simulink model "LQG_test"  (R2015a)
settings: Solver=ode5  StartTime=0.0  StopTime=10  FixedStep=5e-5  RelTol=1e-3
values from neighbouring files (symbols this model uses):
  Ak = [-152.325686755 -1244.77465728 104.064643037 -74.8210490781 -336.947410696 65.1035189281 1409.57049441 -62.9419296076 -9.35522709238 -10.9041878944 -334.481680301 55.3119192038 ... (36 elements, 6x6)]    [controller_reduced.mat]    (also in main_matlab.m = rlqg.A)
  Bk = [0.848659506089 1.67970243216 -36.3236622756 32.4490717083 261.577141309 -45.5608120439]    [controller_reduced.mat]    (also in main_matlab.m = rlqg.B)
  Ck = [6.82372491135  -11.0450495122  -20.4409731276  11.638209929  -14.6880839063  2.898985738; -41.3723172328  25.8226085821  7.60966961308  -0.0537947220508  -9.41528556637  3.11557261268]    [controller_reduced.mat]    (also in main_matlab.m = rlqg.C)
  Dk = [0 0]    [controller_reduced.mat]    (also in main_matlab.m = rlqg.D)
undefined symbols (not defined in the file or in its folder): A, B, C, H
libraries: simulink x1
settings Model: Creator=p4wp4w  LastModifiedBy=Ablah

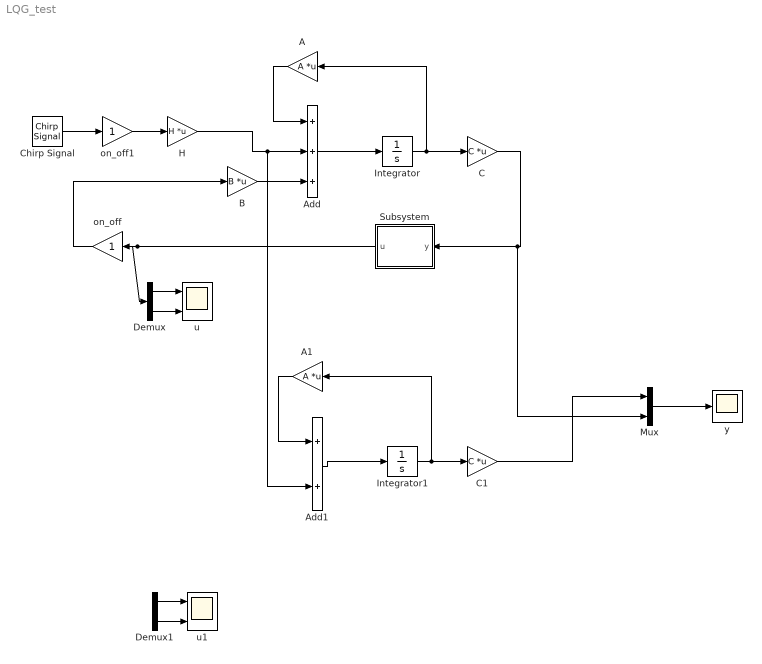
== system LQG_test ==
  A : Gain  Gain=A  Multiplication=Matrix(K*u)
  A1 : Gain  Gain=A  Multiplication=Matrix(K*u)
  Add : Sum  Inputs=+++
  Add1 : Sum
  B : Gain  Gain=B  Multiplication=Matrix(K*u)
  C : Gain  Gain=C  Multiplication=Matrix(K*u)
  C1 : Gain  Gain=C  Multiplication=Matrix(K*u)
  Chirp Signal : simulink/Sources/Chirp Signal  f1=0.1  T=10  f2=240
  Demux : Demux  Outputs=2
  Demux1 : Demux  Outputs=2
  H : Gain  Gain=H  Multiplication=Matrix(K*u)
  Integrator : Integrator
  Integrator1 : Integrator
  Mux : Mux  Inputs=2
  Subsystem : Subsystem
  on_off : Gain
  on_off1 : Gain
  u : Scope  NumInputPorts=2
      settings: YMin=-1.5~-2  YMax=1.5~2
  u1 : Scope  NumInputPorts=2
      settings: YMin=-1.5~-2  YMax=1.5~2  SaveName=ScopeData2
  y : Scope
      settings: YMin=-0.03  YMax=0.03
  wires:
  Add/1 -> Integrator/1
  A/1 -> Add/1
  B/1 -> Add/3
  Integrator/1 -> C/1, A/1
  Chirp Signal/1 -> on_off1/1
  on_off/1 -> B/1
  Demux/1 -> u/1
  Demux/2 -> u/2
  Subsystem/1("u ") -> Demux/1, on_off/1
  on_off1/1 -> H/1
  Add1/1 -> Integrator1/1
  A1/1 -> Add1/1
  Integrator1/1 -> A1/1, C1/1
  Demux1/1 -> u1/1
  Demux1/2 -> u1/2
  H/1 -> Add1/2, Add/2
  C1/1 -> Mux/1
  C/1 -> Mux/2, Subsystem/1(y)
  Mux/1 -> y/1

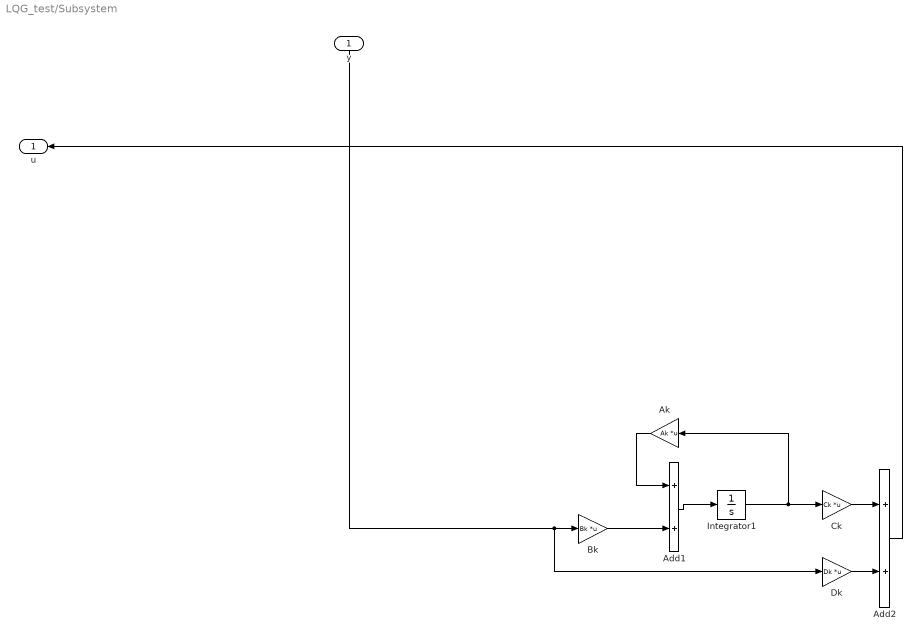
== system LQG_test/Subsystem ==
  y : Inport
  Add1 : Sum
  Add2 : Sum
  Ak : Gain  Gain=Ak  Multiplication=Matrix(K*u)
  Bk : Gain  Gain=Bk  Multiplication=Matrix(K*u)
  Ck : Gain  Gain=Ck  Multiplication=Matrix(K*u)
  Dk : Gain  Gain=Dk  Multiplication=Matrix(K*u)
  Integrator1 : Integrator
  "u " : Outport
  wires:
  y/1 -> Bk/1, Dk/1
  Add2/1 -> "u "/1
  Bk/1 -> Add1/2
  Ak/1 -> Add1/1
  Add1/1 -> Integrator1/1
  Dk/1 -> Add2/2
  Integrator1/1 -> Ck/1, Ak/1
  Ck/1 -> Add2/1
